simulink model "tp2_1"  (R2023b)
settings: Solver=VariableStepAuto  StartTime=0.0  StopTime=10.0  RelTol=1e-3
settings Model: Creator=rusha  LastModifiedBy=rusha

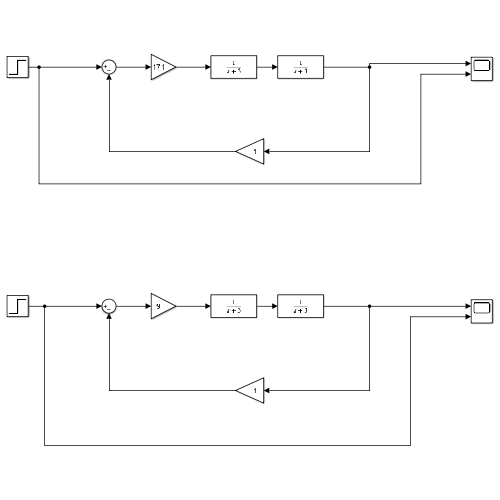
[thumbnail: Simulink's stored preview of the top-level diagram]
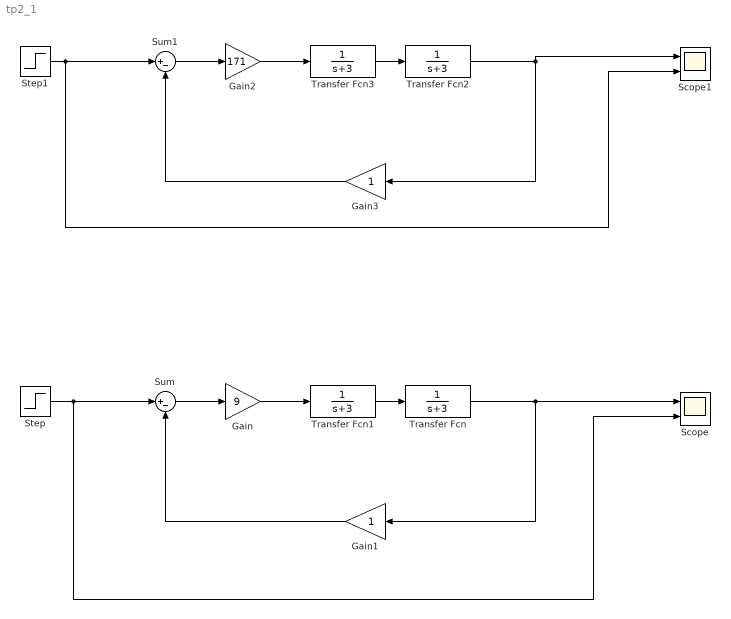
== system tp2_1 ==
  Gain : Gain  Gain=9
  Gain1 : Gain
  Gain2 : Gain  Gain=171
  Gain3 : Gain
  Scope : Scope  NumInputPorts=2
  Scope1 : Scope  NumInputPorts=2
  Step : Step  SampleTime=0
  Step1 : Step  SampleTime=0
  Sum : Sum  Inputs=|+-
  Sum1 : Sum  Inputs=|+-
  Transfer Fcn{,1..3} (4 alike) : TransferFcn  Denominator=[1 3]
  wires:
  Step1/1 -> Scope1/2, Sum1/1
  Transfer Fcn/1 -> Gain1/1, Scope/1
  Transfer Fcn3/1 -> Transfer Fcn2/1
  Sum/1 -> Gain/1
  Transfer Fcn1/1 -> Transfer Fcn/1
  Step/1 -> Scope/2, Sum/1
  Sum1/1 -> Gain2/1
  Transfer Fcn2/1 -> Gain3/1, Scope1/1
  Gain2/1 -> Transfer Fcn3/1
  Gain/1 -> Transfer Fcn1/1
  Gain3/1 -> Sum1/2
  Gain1/1 -> Sum/2
